simulink model "System_Design_Quadrocopter_Dynamics3"  (Simulink 7.4)
settings: Solver=ode45  StartTime=0.0  StopTime=inf  RelTol=1e-3
values from neighbouring files (symbols this model uses):
  K_ret = place(System.a, System.b, [-18 -10 -9 -5 -7])    [Test_Reglerauslegung.m]    (also in auslegung.m = place(System.a, System.b, [-2 -4 -3]))
  KV = KV'    [Reglerauslegung.m]    (also in Test_Reglerauslegung.m; auslegung.m)
  KvPhi = 0.5    [Test_Reglerauslegung.m]
  KvPsi = 0.08    [Test_Reglerauslegung.m]
  KvTheta = 0.4    [Test_Reglerauslegung.m]
undefined symbols (not defined in the file or in its folder): g, m, Ts
libraries: simulink x13, dspobslib x4, Control_lib x2, Copter_Library x1
(part 2 of 2)

== matlab function Control/Embedded PID Control ==
  settings: updateMethod=DISCRETE  sampleTime=0.005
  data: u input double; y output double
function y = fcn(u)
%#eml
persistent e_r_Roll_1 e_Roll_1 r_Roll_I_State r_Roll_Filter_State 
persistent e_r_Pitch_1 e_Pitch_1 r_Pitch_I_State r_Pitch_Filter_State 
persistent e_r_Yaw_1 r_Yaw_I_State r_Yaw_Filter_State
persistent M1_limited M2_limited M3_limited M4_limited 
%  first time initialization
if isempty(M1_limited) 
    M1_limited=uint8(0);
    M2_limited=uint8(0);
    M3_limited=uint8(0);
    M4_limited=uint8(0);
    e_r_Roll_1 = double(0);
    e_Roll_1 = double(0);
    r_Roll_I_State = double(0);
    r_Roll_Filter_State = double(0); 
    e_r_Pitch_1 = double(0);
    e_Pitch_1 = double(0);
    r_Pitch_I_State = double(0); 
    r_Pitch_Filter_State = double(0); 
    e_r_Yaw_1 = double(0); 
    r_Yaw_I_State = double(0); 
    r_Yaw_Filter_State = double(0);
end
IRoll = double(0);
FiltRoll = double(0);
IPitch = double(0);
FiltPitch = double(0);
Ts = 0.005; % sec
G = 9.810; % m/sec²
maxRemotePitch = 128;
maxRemoteRoll = 128;
maxRemoteYaw = 128;
maxPitchAngle = pi/4;
maxRollAngle  = pi/4;
maxYawRate = 200;
sensorSensitivityX = 340;
sensorSensitivityY = 340;
sensorSensitivityZ = 340;
copterState.gyroPOffset = 505;
copterState.gyroROffset = 505;
copterState.gyroYOffset = 505;
copterState.YawRateI_State = 0;
copterState.YawRateD_Filter = 0;
copterState.PitchRateI_State = 0;
copterState.PitchRateD_Filter = 0;
copterState.RollRateI_State = 0;
copterState.RollRateD_Filter = 0;
% copy inputs to variables with easy to know names
copterState.angVelRRaw =  u(3);
copterState.accYRaw = u(2);
copterState.angVelPRaw = u(4);
copterState.accXRaw = u(1);
copterState.accZRaw = 0; %not available
copterState.angVelYRaw = u(5);
copterState.remoteForceRaw = u(9);
copterState.remotePitchRaw = u(7);
copterState.remoteRollRaw = u(6);
copterState.remoteYawRaw = u(8);
copterState.accY = int16(0);
copterState.accX = int16(0);
copterState.accZ = int16(0);
copterState.angP = int16(0);
copterState.angR = int16(0);
copterState.angVelP = int16(0);
copterState.angVelR = int16(0);
copterState.angVelY = int16(0);
copterState.remotePitch = int16(0);
copterState.remoteRoll = int16(0);
copterState.remoteForce = int16(0);
copterState.remoteYaw = int16(0);
angP = double(0);
angR = double(0);

% Convert Data like in the copter
% Accelerometer
%%%%%%%%%%%%%%%%%
  %/* calculate the physical acceleration values in [(10 * m)/(s^2)], as needed by the control algorithm */
  copterState.accY = int16(((int32(copterState.accYRaw) * G) / sensorSensitivityY) / 10);
  copterState.accX = -int16(((int32(copterState.accXRaw) * G) / sensorSensitivityX) / 10);
  copterState.accZ = -int16(((int32(copterState.accZRaw) * G) / sensorSensitivityZ) / 10);
  %// [ 10000*rad ]
  copterState.angP = -int16(int32(copterState.accXRaw)*1000/340);
  copterState.angR = -int16(int32(copterState.accYRaw)*1000/340);
  
  % Gyroscopes [100 * rad/sec]
  %%%%%%%%%%%%%%
   copterState.angVelP     = -int16(double(copterState.angVelPRaw-copterState.gyroPOffset) * 0.938349);
   copterState.angVelR     = int16(double(copterState.angVelRRaw-copterState.gyroROffset) * 0.938349);
   copterState.angVelY     = -int16(double(copterState.angVelYRaw-copterState.gyroYOffset) * 0.938349);
   
   % Remote
   %%%%%%%%%%%%%
  copterState.remotePitch    = int16(maxPitchAngle*int32(copterState.remotePitchRaw-128)/maxRemotePitch);
  copterState.remoteRoll     = -int16(maxRollAngle*int32(copterState.remoteRollRaw-128)/maxRemoteRoll);
  copterState.remoteForce    = int16(copterState.remoteForceRaw); 
  copterState.remoteYaw      = int16(maxYawRate*int32(copterState.remoteYawRaw-128)/maxRemoteYaw);

% Set outputs to Values calculated last sample time
y = double([M1_limited;M2_limited;M3_limited;M4_limited]);
   
   angP = double(copterState.angP)/1000;
   angR = double(copterState.angR)/1000;
   
% calculate error values for the controlled angles
   % Pitch error 
   e_Pitch = double(copterState.remotePitch) - angP;
   % Roll error
   e_Roll = double(copterState.remoteRoll) - angR;
   % calculate controller output for the angles (I State & FilterState are not necessary cause only p is used
   [m_Roll, IRoll, FiltRoll] = PID(150,0.5,0,0,e_Roll,e_Roll_1,IRoll, FiltRoll, Ts);
   [m_Pitch, IPitch, FiltPitch] = PID(150,0.5,0,0,e_Pitch,e_Pitch_1,IPitch,FiltPitch,Ts);
      
   % Yaw Rate error
   e_r_Yaw = double(copterState.remoteYaw) - double(copterState.angVelY);
   % Pitch Rate error
   e_r_Pitch = m_Pitch - double(copterState.angVelP);
   % Roll Rate error
   e_r_Roll = m_Roll - double(copterState.angVelR);
   % calculate  controller output for rates
   [m_r_Yaw,r_Yaw_I_State, r_Yaw_Filter_State] = PID (70, ...
       0.5, 0,0,e_r_Yaw, e_r_Yaw_1, r_Yaw_I_State, r_Yaw_Filter_State,Ts);
   [m_r_Roll,r_Roll_I_State, r_Roll_Filter_State] = PID (70, ...
       0.5, 0,0,e_r_Roll, e_r_Roll_1, r_Roll_I_State, r_Roll_Filter_State,Ts);
   [m_r_Pitch,r_Pitch_I_State, r_Pitch_Filter_State] = PID (70, ...
       0.5, 0,0,e_r_Pitch, e_r_Pitch_1, r_Pitch_I_State, r_Pitch_Filter_State,Ts);
   
   % save error for next sample time
   e_Roll_1 = e_Roll;
   e_Pitch_1 = e_Pitch;
   e_r_Roll_1 = e_r_Roll;
   e_r_Pitch_1 = e_r_Pitch;
   e_r_Yaw_1 = e_r_Yaw;
 
   %//Calculate new setpoints of all motors
    M1 = (copterState.remoteForce-m_r_Pitch+m_r_Yaw);
    M2 = (copterState.remoteForce+m_r_Roll-m_r_Yaw);
    M3 = (copterState.remoteForce+m_r_Pitch+m_r_Yaw);
    M4 = (copterState.remoteForce-m_r_Roll-m_r_Yaw);
   
   
    %// saturate setpoint of motor1 to 0 if less and 255 if above
    if M1 < 0
      M1_limited = uint8(0);
    else
        if M1 > 255
            M1_limited = uint8(255); 
        else
            M1_limited=uint8(M1);
        end
    end
    
    %// saturate setpoint of motor2 to 0 if less and 255 if above
    if M2 < 0
      M2_limited = uint8(0);
    else
        if M2 > 255
          M2_limited = uint8(255); 
        else
          M2_limited=uint8(M2);
        end
    end

    %// saturate setpoint of motor3 to 0 if less and 255 if above
  if M3 < 0
      M3_limited = uint8(0);
  else
      if M3 > 255
        M3_limited = uint8(255); 
      else
         M3_limited=uint8(M3);
      end
  end
    
    %// saturate setpoint of motor4 to 0 if less and 255 if above
    if M4 < 0
      M4_limited = uint8(0);
    else
        if M4 > 255
           M4_limited = uint8(255); 
        else
           M4_limited=uint8(M4);
        end
    end

% This function calculates the next Value of the ?ideal? PID controller
function [ret, I_State, Filt_State] = PID (P, I, D, N, ek, ek_1, I_State, Filt_State, Ts)

if P ~= 0 
    if I ~= 0
        % calculate new itegral value
        I_State = ek * Ts * I + I_State;
    else
        I_State = 0;
    end

    if D ~= 0
        % calculate new derivative Value
        yd = (ek - ek_1)/Ts * D;

        % Filter the derivative  Value
        Filt_State = Ts * (yd -N*Filt_State)+ Filt_State ;
    else
        Filt_State = 0;
    end

    % Add all values and multiply P gain to all
    ret = (P * ek + I_State + Filt_State);

else
    ret = 0;
end


function ret16 = mult_fp (A, B, factor)
    ret32 = int32(A) * int32(B)/factor;
    if ret32 > 2^15-1
        ret16 = int16(2^15-1);
    else
        if ret32 < -2^15+1
            ret16 = int16(-2^15+1);
        else
            ret16 = int16(ret32);
        end
    end
% end of mult_fp    

function ret16 = div_fp(A, B, factor)
if B == 0
    display('divide by ZERO !!!!')
    ret16 = 2^16-1;
else
    ret32 = int32(A)*factor/int32(B);
     if ret32 > 2^15-1
        ret16 = int16(2^15-1);
    else
        if ret32 < -2^15+1
            ret16 = int16(-2^15+1);
        else
            ret16 = int16(ret32);
        end
    end
end
% end of div_fp
